simulink model "proj_simscape"  (R2015a)
settings: Solver=ode3  StartTime=0.0  StopTime=3  FixedStep=0.01  RelTol=1e-3
undefined symbols (not defined in the file or in its folder): Bj, Bp, Kr, Mj, Mp
settings Model: Creator=ahmed alaa  LastModifiedBy=ahmed alaa

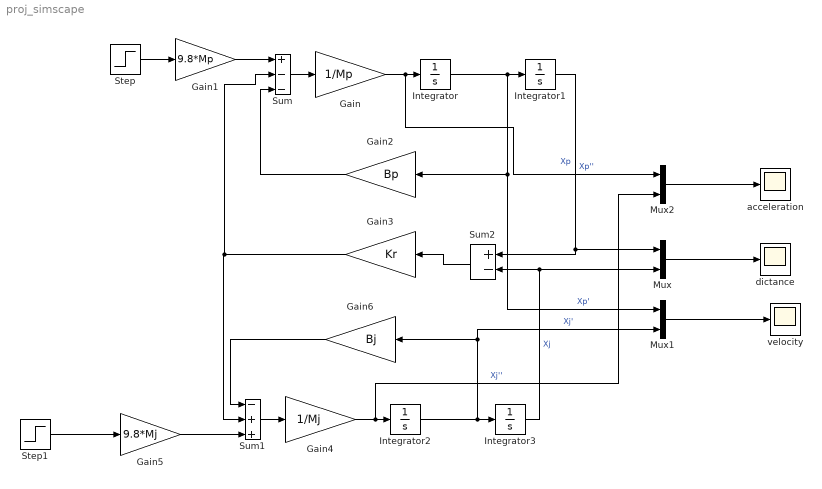
== system proj_simscape ==
  Gain : Gain  Gain=1/Mp
  Gain1 : Gain  Gain=9.8*Mp
  Gain2 : Gain  Gain=Bp
  Gain3 : Gain  Gain=Kr
  Gain4 : Gain  Gain=1/Mj
  Gain5 : Gain  Gain=9.8*Mj
  Gain6 : Gain  Gain=Bj
  Integrator : Integrator  InitialCondition=20
  Integrator1 : Integrator
  Integrator2 : Integrator  InitialCondition=20
  Integrator3 : Integrator
  Mux : Mux  Inputs=2
  Mux1 : Mux  Inputs=2
  Mux2 : Mux  Inputs=2
  Step : Step  Time=0  SampleTime=0
  Step1 : Step  Time=0  SampleTime=0
  Sum : Sum  Inputs=+--
  Sum1 : Sum  Inputs=-++
  Sum2 : Sum  Inputs=+-
  "acceleration " : Scope
      settings: SaveName=ScopeData2
  dictance : Scope
  velocity : Scope
  wires:
  Integrator/1 -> Mux1/1, Gain2/1, Integrator1/1  "Xp'"
  Gain/1 -> Mux2/1, Integrator/1  "Xp''"
  Sum/1 -> Gain/1
  Step/1 -> Gain1/1
  Gain1/1 -> Sum/1
  Gain2/1 -> Sum/3
  Gain3/1 -> Sum/2, Sum1/2
  Integrator2/1 -> Integrator3/1, Mux1/2, Gain6/1  "Xj'"
  Gain4/1 -> Mux2/2, Integrator2/1  "Xj''"
  Sum1/1 -> Gain4/1
  Step1/1 -> Gain5/1
  Gain5/1 -> Sum1/3
  Gain6/1 -> Sum1/1
  Integrator1/1 -> Mux/1, Sum2/1  "Xp"
  Integrator3/1 -> Mux/2, Sum2/2  "Xj"
  Sum2/1 -> Gain3/1
  Mux/1 -> dictance/1
  Mux1/1 -> velocity/1
  Mux2/1 -> "acceleration "/1
